simulink model "Regulador_discreto_plantilla"  (R2016a)
settings: Solver=VariableStepAuto  StartTime=0.0  StopTime=10.0  RelTol=1e-3
values from neighbouring files (symbols this model uses):
  k_dis = place(A_dis,B_dis,Pol_des_dis)    [Regulador_seguidor_observador_codigo.m]
  tm = 0.1    [Regulador_seguidor_observador_codigo.m]
undefined symbols (not defined in the file or in its folder): A_dis, B_dis, C_dis
settings Model: Creator=Daniel  LastModifiedBy=Daniel

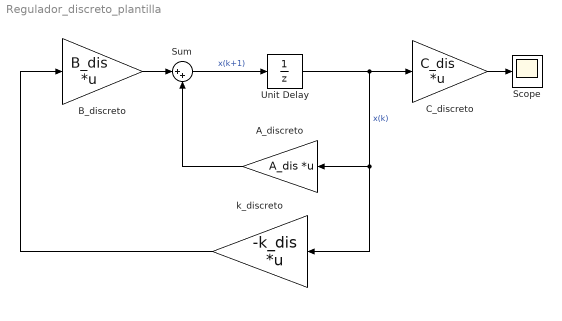
== system Regulador_discreto_plantilla ==
  A_discreto : Gain  Gain=A_dis  Multiplication=Matrix(K*u) (u vector)
  B_discreto : Gain  Gain=B_dis  Multiplication=Matrix(K*u) (u vector)
  C_discreto : Gain  Gain=C_dis  Multiplication=Matrix(K*u) (u vector)
  Scope : Scope
  Sum : Sum  Inputs=|++
  Unit Delay : UnitDelay  InitialCondition=[1;1]  SampleTime=tm
  k_discreto : Gain  Gain=-k_dis  Multiplication=Matrix(K*u) (u vector)
  wires:
  Unit Delay/1 -> k_discreto/1, A_discreto/1, C_discreto/1  "x(k)"
  A_discreto/1 -> Sum/2
  Sum/1 -> Unit Delay/1  "x(k+1)"
  C_discreto/1 -> Scope/1
  k_discreto/1 -> B_discreto/1
  B_discreto/1 -> Sum/1
